simulink model "model_of_sous_vide"  (R2021b)
settings: Solver=VariableStepAuto  StartTime=0.0  StopTime=3600.0  RelTol=1e-3
values from neighbouring files (symbols this model uses):
  A = 0.07    [setup_values.m]
  a = 50    [setup_values.m]
  c = 4180    [setup_values.m]
  Ki = 10    [setup_values.m]
  Kp = 10    [setup_values.m]
  m = 2    [setup_values.m]
  P = 300    [setup_values.m]
  Sp = 82    [setup_values.m]
  Ta = 19    [setup_values.m]
  Ts = 1    [setup_values.m]
settings Model: Creator=felixmalmsjo  LastModifiedBy=felixmalmsjo

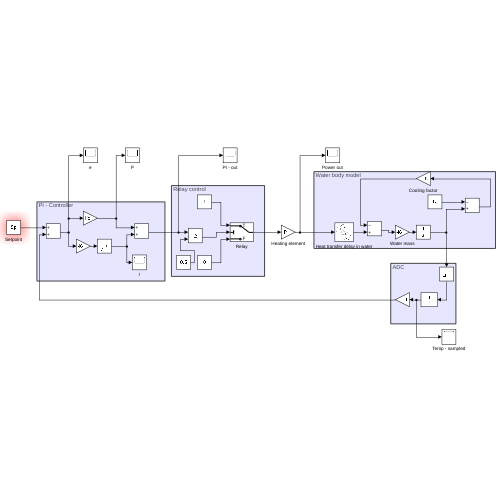
[thumbnail: Simulink's stored preview of the top-level diagram]
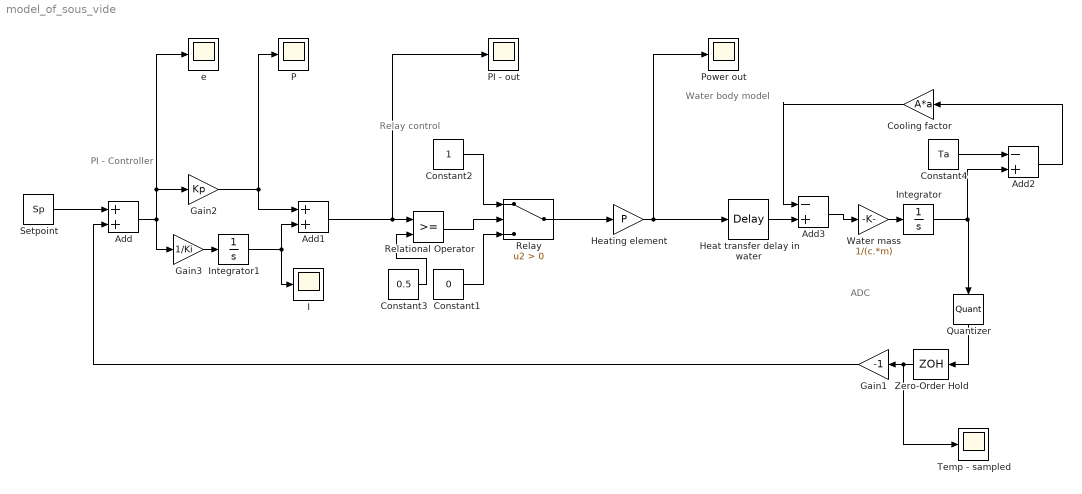
== system model_of_sous_vide ==
  note: ADC
  note: Water body model
  note: Relay control
  note: PI - Controller
  Add : Sum
  Add1 : Sum
  Add2 : Sum  Inputs=-+
  Add3 : Sum  Inputs=-+
  Constant1 : Constant  Value=0
  Constant2 : Constant
  Constant3 : Constant  Value=0.5
  Constant4 : Constant  Value=Ta
  Cooling factor : Gain  Gain=A*a
  Gain1 : Gain  Gain=-1
  Gain2 : Gain  Gain=Kp
  Gain3 : Gain  Gain=1/Ki
  Heat transfer delay in water : TransportDelay
  Heating element : Gain  Gain=P
  I : Scope
  Integrator : Integrator  InitialCondition=Ta
  Integrator1 : Integrator  LimitOutput=on  UpperSaturationLimit=1  LowerSaturationLimit=-1
  P : Scope
  PI - out : Scope
  Power out : Scope
  Quantizer : Quantizer  QuantizationInterval=Td
  Relational Operator : RelationalOperator  OutDataTypeStr=boolean  RndMeth=Simplest
  Relay : Switch  Criteria=u2 > Threshold
  Setpoint : Constant  Value=Sp
  Temp - sampled : Scope
  Water mass : Gain  Gain=1/(c.*m)
  Zero-Order Hold : ZeroOrderHold  SampleTime=Ts
  e : Scope
  wires:
  Water mass/1 -> Integrator/1
  Integrator/1 -> Quantizer/1, Add2/2
  Setpoint/1 -> Add/1
  Gain1/1 -> Add/2
  Add/1 -> Gain3/1, e/1, Gain2/1
  Gain3/1 -> Integrator1/1
  Gain2/1 -> P/1, Add1/1
  Integrator1/1 -> Add1/2, I/1
  Add1/1 -> Relational Operator/1, PI - out/1
  Relational Operator/1 -> Relay/2
  Constant1/1 -> Relay/3
  Constant2/1 -> Relay/1
  Relay/1 -> Heating element/1
  Constant3/1 -> Relational Operator/2
  Heating element/1 -> Power out/1, Heat transfer delay in water/1
  Constant4/1 -> Add2/1
  Heat transfer delay in water/1 -> Add3/2
  Add3/1 -> Water mass/1
  Add2/1 -> Cooling factor/1
  Cooling factor/1 -> Add3/1
  Zero-Order Hold/1 -> Temp - sampled/1, Gain1/1
  Quantizer/1 -> Zero-Order Hold/1
